simulink model "test_2"  (R2022a)
settings: Solver=ode4  StartTime=0.0  StopTime=50  FixedStep=0.01  RelTol=1e-3
libraries: simulink x1
settings Model: Creator=Alireza Sharifi  LastModifiedBy=Alireza Sharifi

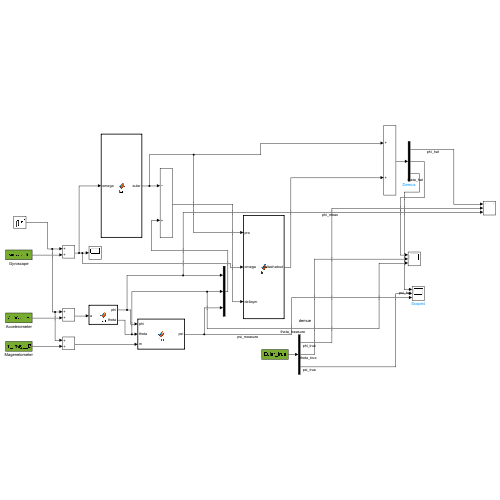
[thumbnail: Simulink's stored preview of the top-level diagram]
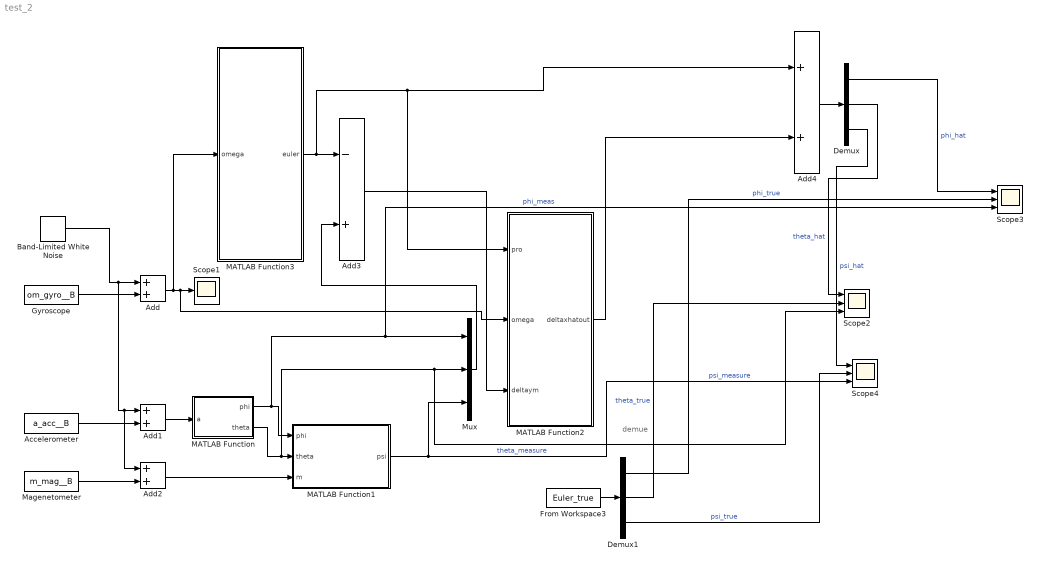
== system test_2 ==
  note: demue
  Accelerometer : FromWorkspace  VariableName=a_acc__B  SampleTime=0.01
  Add{,1..2,4} (4 alike) : Sum
  Add3 : Sum  Inputs=-+
  Band-Limited White Noise : simulink/Sources/Band-Limited White Noise  Cov=1e-5  Ts=0.01  seed=[23341]
  Demux : Demux  Outputs=3
  Demux1 : Demux  Outputs=3
  From Workspace3 : FromWorkspace  VariableName=Euler_true  SampleTime=0.01
  Gyroscope : FromWorkspace  VariableName=om_gyro__B  SampleTime=0.01
  MATLAB Function : MATLAB Function  TreatAsAtomicUnit=on
  MATLAB Function1 : MATLAB Function  TreatAsAtomicUnit=on
  MATLAB Function2 : MATLAB Function  TreatAsAtomicUnit=on
  MATLAB Function3 : MATLAB Function  TreatAsAtomicUnit=on
  Magenetometer : FromWorkspace  VariableName=m_mag__B  SampleTime=0.01
  Mux : Mux  Inputs=3
  Scope1 : Scope
  Scope2 : Scope  NumInputPorts=3
  Scope3 : Scope  NumInputPorts=3
  Scope4 : Scope  NumInputPorts=3
  wires:
  Gyroscope/1 -> Add/2
  Add/1 -> MATLAB Function3/1(omega), MATLAB Function2/2(omega), Scope1/1
  Accelerometer/1 -> Add1/2
  Magenetometer/1 -> Add2/2
  Band-Limited White Noise/1 -> Add2/1, Add1/1, Add/1
  Add1/1 -> MATLAB Function/1(a)
  Add2/1 -> MATLAB Function1/3(m)
  MATLAB Function/2(theta) -> Scope2/3, Mux/2, MATLAB Function1/2(theta)  "theta_measure"
  MATLAB Function/1(phi) -> Scope3/3, Mux/1, MATLAB Function1/1(phi)  "phi_meas"
  MATLAB Function1/1(psi) -> Scope4/3, Mux/3  "psi_measure"
  MATLAB Function2/1(deltaxhatout) -> Add4/2
  Demux/1 -> Scope3/1  "phi_hat"
  Demux/2 -> Scope2/1  "theta_hat"
  Demux/3 -> Scope4/1  "psi_hat"
  From Workspace3/1 -> Demux1/1
  Demux1/2 -> Scope2/2  "theta_true"
  Demux1/1 -> Scope3/2  "phi_true"
  Demux1/3 -> Scope4/2  "psi_true"
  MATLAB Function3/1(euler) -> Add4/1, MATLAB Function2/1(pro), Add3/1
  Mux/1 -> Add3/2
  Add3/1 -> MATLAB Function2/3(deltaym)
  Add4/1 -> Demux/1

== matlab function test_2/MATLAB Function1 ==
  data: phi input; psi output; theta input; m input
function psi = fcn(phi,theta,m)
mx=m(1);
my=m(2);
mz=m(3);
%
num_psi=-cos(phi)*my+sin(phi)*mz;
den_psi=cos(theta)*mx+sin(theta)*sin(phi)*my+sin(theta)*cos(phi)*mz;
declination_angle=-4.0266*pi/180;
psi=atan2(num_psi,den_psi)+declination_angle;

== matlab function test_2/MATLAB Function ==
  data: a input; phi output; theta output
function [phi,theta] = fcn(a)
ax=a(1);
ay=a(2);
az=a(3);
g=9.81;
phi=atan2(-ay,-az);
theta=asin(ax/g);

== matlab function test_2/MATLAB Function2 ==
  data: pro input; omega input; deltaxhatout output; deltaym input
function deltaxhatout = fcn(pro,omega,deltaym)
phi=pro(1);
theta=pro(2);
psi=pro(3);
p=omega(1);
q=omega(2);
r=omega(3);
%%
persistent deltaxhat P
if isempty(deltaxhat)
    deltaxhat=[0;0;0];
end
if isempty(P)
    P=[100 0 0;
        0  100 0;
        0  0   100];
end
%%
Ts=0.01;
Q=[1 0 0;
        0  1 0;
        0  0   1];
R=0.01*[1 0 0;
        0  1 0;
        0  0   1];
%%
F=[1+Ts*tan(theta)*(q*cos(phi)-r*sin(phi)) ...
    Ts*(q*sin(phi)+r*cos(phi))/(cos(theta)^2) 0;
  Ts*(-q*sin(phi)-r*cos(phi))   1   0;
  Ts*(q*cos(phi)-r*sin(phi))/cos(theta) ...
     Ts*sin(theta)*(q*sin(phi)+r*cos(phi))/(cos(theta)^2) 1];
deltaxhat=F*deltaxhat;
%%
%%
Gama=[Ts Ts*tan(theta)*sin(phi) Ts*tan(theta)*cos(phi);
    0  Ts*cos(phi)  -Ts*sin(phi);
    0  Ts*sin(phi)/cos(theta) Ts*cos(phi)/cos(theta)];
P=F*P*F'+Gama*Q*Gama';
%%
C=[1 0 0;
    0 1 0;
    0 0 1];
deltayhat=C*deltaxhat;
K=P*C'*inv(C*P*C'+R);
deltaxhat=deltaxhat+K*(deltaym-deltayhat);
P=(eye(3)-K*C)*P*(eye(3)-K*C)'+K*R*K';
deltaxhatout=deltaxhat;

== matlab function test_2/MATLAB Function3 ==
  data: omega input; euler output
function euler = fcn(omega)
p=omega(1);
q=omega(2);
r=omega(3);
%%
persistent xhat
if isempty(xhat)
    xhat=[0;0;0];
end
Ts=0.01;
phi=xhat(1);
theta=xhat(2);
psi=xhat(3);
xhat1=phi+Ts*(p+tan(theta)*sin(phi)*q+r*cos(phi)*tan(theta));
xhat2=theta+Ts*(q*cos(phi)-r*sin(phi));
xhat3=psi+Ts*(sec(theta)*(q*sin(phi)+r*cos(phi)));
%%
xhat=[xhat1;xhat2;xhat3];
euler=xhat;
